simulink model "IGM_3D_MP"  (R2021a)
settings: Solver=VariableStepAuto  StartTime=0.0  StopTime=1000  RelTol=1e-3
values from neighbouring files (symbols this model uses):
  X0 = [x0;y0;z0;vx0;vy0;vz0]    [Main.m]
undefined symbols (not defined in the file or in its folder): p
settings Model: Creator=FawadFarooq  LastModifiedBy=FawadFarooq

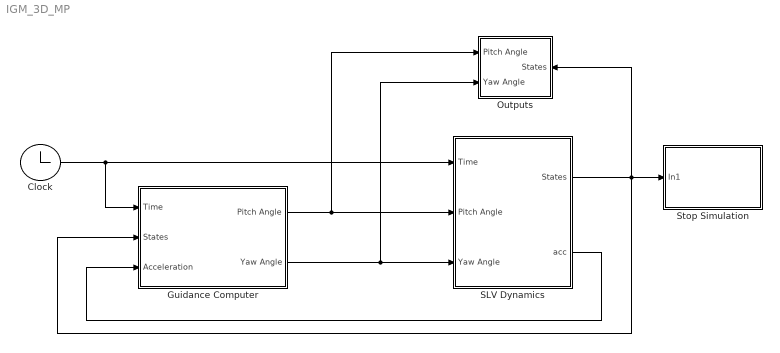
== system IGM_3D_MP ==
  Clock : Clock
  Guidance Computer : Subsystem
  Outputs : Subsystem
      settings: PortSchema="{\"entries\":[{\"content\":{\"sides\":[{\"content\":{\"connectorIds\":[\"In1\",\"In2\"]},\"type\":\"ConnectorPlacement.EquallySpacedRectSide\",\"uuid\":\"072ea4b5-769e-43eb-a3c3-6af6f3856208\"},{\"content\":{\"connectorIds\":[\"In3\"],\"side\":\"RIGHT\"},\"type\":\"ConnectorPlacement.EquallySpacedRectSide\",\"uuid\":\"64728ef0-65f2-4c87-b895-8041e6a7d13d\"},{\"content\":{\"connectorIds\":[],\"side\":\"TOP\"},\"type\":\"ConnectorPlacement.EquallySpacedRectSide\",\"uuid\":\"9708094a-022a-48f5-847a-dae2381fa515\"}]},\"type\":\"ConnectorPlacement.EquallySpacedConnector\",\"uuid\":\"193dd09d-2000-471e-91a9-709041d894d9\"}],\"packageUris\":[\"http://schema.mathworks.com/mf0/Connector/R2020b\"],\"version\":\"1.0\"}"
  SLV Dynamics : Subsystem
  Stop Simulation : Subsystem
  wires:
  Clock/1 -> Guidance Computer/1(Time), SLV Dynamics/1(Time)
  SLV Dynamics/1(States) -> Outputs/3(States), Stop Simulation/1(In1), Guidance Computer/2(States)
  Guidance Computer/2(Yaw Angle) -> Outputs/2(Yaw Angle), SLV Dynamics/3(Yaw Angle)
  Guidance Computer/1(Pitch Angle) -> Outputs/1(Pitch Angle), SLV Dynamics/2(Pitch Angle)
  SLV Dynamics/2(acc) -> Guidance Computer/3(Acceleration)

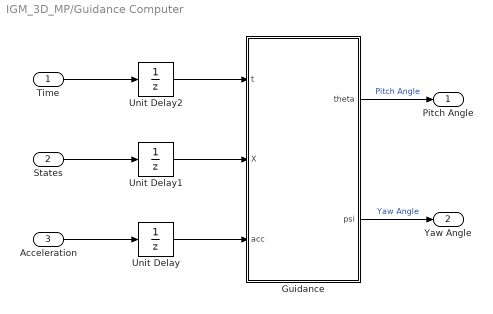
== system IGM_3D_MP/Guidance Computer ==
  Time : Inport
  States : Inport  Port=2
  Acceleration : Inport  Port=3
  Guidance : MATLAB Function  TreatAsAtomicUnit=on  SystemSampleTime=p.Tsamp
  Unit Delay : UnitDelay  InitialCondition=p.Thr3a/p.m03a  SampleTime=-1  HasFrameUpgradeWarning=on
  Unit Delay1 : UnitDelay  InitialCondition=X0  SampleTime=-1  HasFrameUpgradeWarning=on
  Unit Delay2 : UnitDelay  InitialCondition=p.Tsamp  SampleTime=-1  HasFrameUpgradeWarning=on
  Pitch Angle : Outport
  Yaw Angle : Outport  Port=2
  wires:
  Guidance/1(theta) -> Pitch Angle/1  "Pitch Angle"
  Unit Delay2/1 -> Guidance/1(t)
  Unit Delay/1 -> Guidance/3(acc)
  Acceleration/1 -> Unit Delay/1
  Unit Delay1/1 -> Guidance/2(X)
  Guidance/2(psi) -> Yaw Angle/1  "Yaw Angle"
  States/1 -> Unit Delay1/1
  Time/1 -> Unit Delay2/1

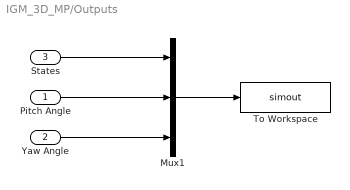
== system IGM_3D_MP/Outputs ==
  Pitch Angle : Inport
  Yaw Angle : Inport  Port=2
  States : Inport  Port=3
  Mux1 : Mux  Inputs=3
  To Workspace : ToWorkspace  VariableName=simout  SaveFormat=Timeseries  SampleTime=-1
  wires:
  States/1 -> Mux1/1
  Mux1/1 -> To Workspace/1
  Pitch Angle/1 -> Mux1/2
  Yaw Angle/1 -> Mux1/3

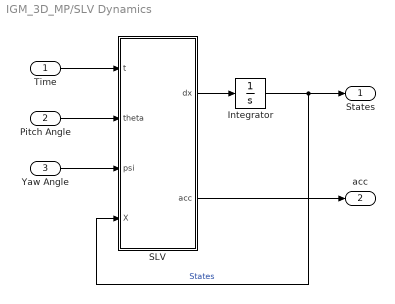
== system IGM_3D_MP/SLV Dynamics ==
  Time : Inport
  Pitch Angle : Inport  Port=2
  Yaw Angle : Inport  Port=3
  Integrator : Integrator  InitialCondition=X0
  SLV : MATLAB Function  TreatAsAtomicUnit=on
  States : Outport
  acc : Outport  Port=2
  wires:
  SLV/1(dx) -> Integrator/1
  Time/1 -> SLV/1(t)
  Integrator/1 -> States/1, SLV/4(X)  "States"
  Yaw Angle/1 -> SLV/3(psi)
  Pitch Angle/1 -> SLV/2(theta)
  SLV/2(acc) -> acc/1

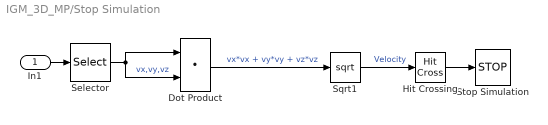
== system IGM_3D_MP/Stop Simulation ==
  In1 : Inport
  Dot Product : DotProduct  InputSameDT=on  OutDataTypeStr=Inherit: Inherit via internal rule
  Hit Crossing : HitCross  HitCrossingOffset=p.vf  HitCrossingDirection=rising
  Selector : Selector  InputPortWidth=6  IndexOptions=Index vector (dialog)  Indices=[4 5 6]  OutputSizes=1
  Sqrt1 : Sqrt  SaturateOnIntegerOverflow=on
  Stop Simulation : Stop
  wires:
  Hit Crossing/1 -> Stop Simulation/1
  In1/1 -> Selector/1
  Selector/1 -> Dot Product/2, Dot Product/1  "vx,vy,vz"
  Dot Product/1 -> Sqrt1/1  "vx*vx + vy*vy + vz*vz"
  Sqrt1/1 -> Hit Crossing/1  "Velocity"

== matlab function IGM_3D_MP/Guidance Computer/Guidance ==
  settings: updateMethod=DISCRETE  sampleTime=0.02
  data: t input; theta output; psi output; X input; acc input; p parameter
function [theta,psi] = fcn(t, X, acc, p) %#ok<*INUSL>

[theta,psi] = igm_3d_mp(t, X, acc, p);

== matlab function IGM_3D_MP/SLV Dynamics/SLV ==
  data: t input; theta input; dx output; psi input; X input; acc output; p parameter
function [dx,acc] = fcn(t,theta,psi,X,p)

u = [cosd(theta)*cosd(psi);
    sind(theta)*cosd(psi);
    sind(psi)];

if (t <= p.tb3a)
    
    mass = p.m03a - p.mdot3a*t; 
    acc = p.Thr3a / mass;
    
elseif (t <= (p.tb3a+p.tc))
    
    mass = p.m0c - p.mdotc*(t-p.tb3a);
    acc = p.Thrc/mass;
    
else
    
    mass = p.m03b - p.mdot3b*(t-(p.tb3a+p.tc));
    acc = p.Thr3b/mass;
    
end

r = norm([X(1);X(2);X(3)]);

rdot = [X(4);
        X(5);
        X(6)];

vdot = acc*u - (p.GM/r^3)*[X(1);X(2);X(3)];

dx = [rdot;vdot];
